simulink library "ElectricSystem"  (R2013a)
settings: Solver=ode3  StartTime=0.0  StopTime=10.0  RelTol=1e-3
settings Model: Creator=torstebo  LastModifiedBy=torstebo

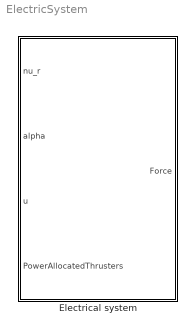
== system ElectricSystem ==
  Electrical system : Subsystem  Tag=electricSystem

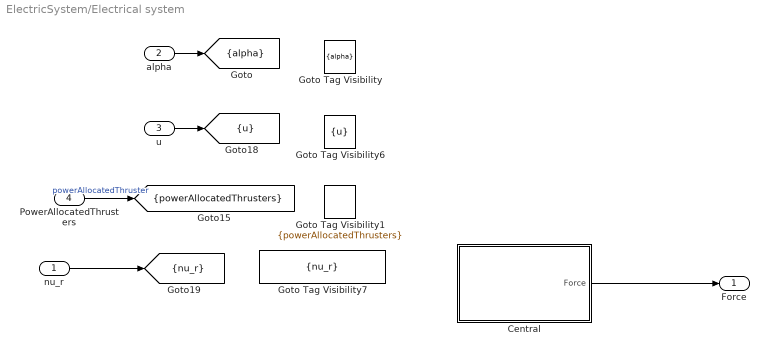
== system ElectricSystem/Electrical system ==
  nu_r : Inport  OutDataTypeStr=double
  alpha : Inport  Port=2  OutDataTypeStr=double
  u : Inport  Port=3  OutDataTypeStr=double
  PowerAllocatedThrusters : Inport  Port=4
  Central : Subsystem
  Goto Tag Visibility : GotoTagVisibility  GotoTag=alpha
  Goto Tag Visibility1 : GotoTagVisibility  GotoTag=powerAllocatedThrusters
  Goto Tag Visibility6 : GotoTagVisibility  GotoTag=u
  Goto Tag Visibility7 : GotoTagVisibility  GotoTag=nu_r
  Force : Outport  OutDataTypeStr=double
  tag scope: alpha=scoped, nu_r=scoped, powerAllocatedThrusters=scoped, u=scoped
  wires:
  alpha/1 -> [alpha]
  u/1 -> [u]
  nu_r/1 -> [nu_r]
  PowerAllocatedThrusters/1 -> [powerAllocatedThrusters]  "powerAllocatedThruster"
  Central/1(Force) -> Force/1

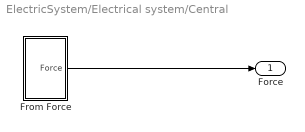
== system ElectricSystem/Electrical system/Central ==
  From Force : Subsystem  Tag=ForceFrom
  Force : Outport  Tag=ForceFrom  OutDataTypeStr=double
  wires:
  From Force/1(Force) -> Force/1

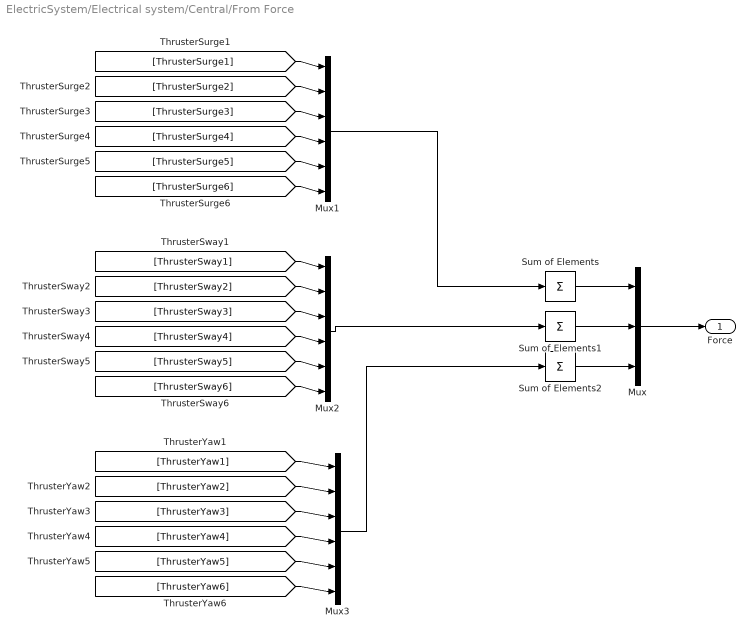
== system ElectricSystem/Electrical system/Central/From Force ==
  Mux : Mux  Inputs=3
  Mux1 : Mux  Tag=ForceFrom/SurgeMerger  Inputs=6
  Mux2 : Mux  Tag=ForceFrom/SwayMerger  Inputs=6
  Mux3 : Mux  Tag=ForceFrom/YawMerger  Inputs=6
  Sum of Elements : Sum  Inputs=+
  Sum of Elements1 : Sum  Inputs=+
  Sum of Elements2 : Sum  Inputs=+
  Force : Outport
  wires:
  Sum of Elements2/1 -> Mux/3
  Sum of Elements/1 -> Mux/1
  Sum of Elements1/1 -> Mux/2
  Mux/1 -> Force/1
  Mux1/1 -> Sum of Elements/1
  Mux2/1 -> Sum of Elements1/1
  Mux3/1 -> Sum of Elements2/1
  [ThrusterSurge1] -> Mux1/1
  [ThrusterSway1] -> Mux2/1
  [ThrusterYaw1] -> Mux3/1
  [ThrusterSurge2] -> Mux1/2
  [ThrusterSway2] -> Mux2/2
  [ThrusterYaw2] -> Mux3/2
  [ThrusterSurge3] -> Mux1/3
  [ThrusterSway3] -> Mux2/3
  [ThrusterYaw3] -> Mux3/3
  [ThrusterSurge4] -> Mux1/4
  [ThrusterSway4] -> Mux2/4
  [ThrusterYaw4] -> Mux3/4
  [ThrusterSurge5] -> Mux1/5
  [ThrusterSway5] -> Mux2/5
  [ThrusterYaw5] -> Mux3/5
  [ThrusterSurge6] -> Mux1/6
  [ThrusterSway6] -> Mux2/6
  [ThrusterYaw6] -> Mux3/6
